simulink model "Yaw_EV_4WD"  (Simulink 8.8)
settings: Solver=ode45  StartTime=0  StopTime=10  FixedStep=0.002  RelTol=1e-3  AbsTol=1e-6
libraries: Solver_SF x1
settings Model: Creator=ywata  LastModifiedBy=mkhan  ExtModeTrigMode=oneshot  ExtModeArmWhenConnect=off
settings DataIOCC: LimitDataPoints=off  SignalLoggingName=sigsOut
settings OptimizationCC: BooleanDataType=off  ExpressionDepthLimit=2147483647
settings DebuggingCC: SaveWithParameterizedLinksMsg=none  SignalResolutionControl=TryResolveAllWithWarning  MultiTaskDSMMsg=warning  MultiTaskCondExecSysMsg=none  SFExecutionAtInitializationDiag=warning
settings HardwareCC: TargetUnknown=on
settings RTWCC: TemplateMakefile=grt_vc.tmf
settings ConfigComp: CovSFcnEnable=off

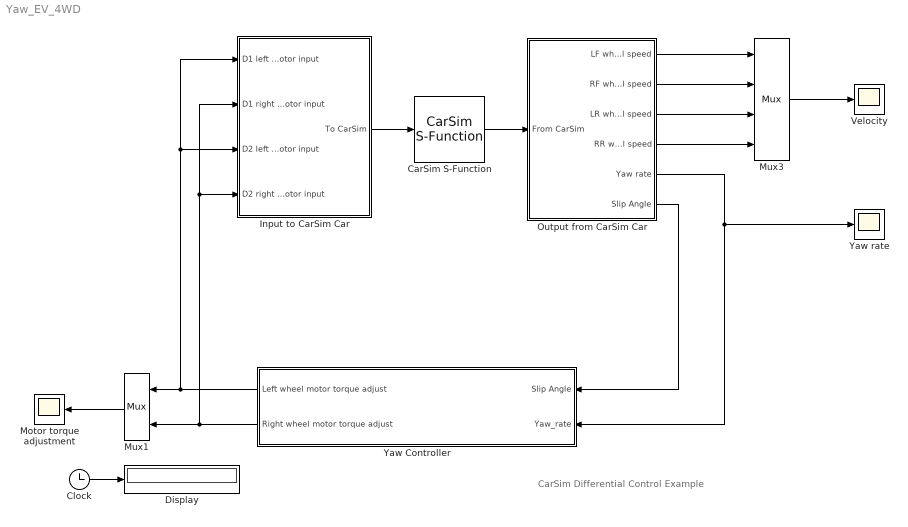
== system Yaw_EV_4WD ==
  note: CarSim Differential Control Example
  CarSim S-Function : Solver_SF/CarSim S-Function  Priority=1  SIMFILE=simfile.sim  Run_RTs=off  vs_state_ind=Run  StopMode_ind=Vehicle Model
  Clock : Clock
  Display : Display
      settings: Format=bank  Decimation=100
  Input to CarSim Car : Subsystem
  Motor torque adjustment : Scope
  Mux1 : Mux  Inputs=2
  Mux3 : Mux
  Output from CarSim Car : Subsystem
  Velocity : Scope
  Yaw Controller : Subsystem  mask{YAW=0.06, CONTROL=25, MAX_TORQUE=300}
      mask prompts: YAW "Yaw Control Gain (-)"; CONTROL "Control Gain (-)"; MAX_TORQUE "Maximum control torque (N)"
  Yaw rate : Scope
  wires:
  CarSim S-Function/1 -> Output from CarSim Car/1(From CarSim)
  Input to CarSim Car/1(To CarSim) -> CarSim S-Function/1
  Yaw Controller/1(Left wheel motor torque adjust) -> Mux1/1, Input to CarSim Car/3(D2 left motor input), Input to CarSim Car/1(D1 left motor input)
  Yaw Controller/2(Right wheel motor torque adjust) -> Input to CarSim Car/2(D1 right motor input), Input to CarSim Car/4(D2 right motor input), Mux1/2
  Clock/1 -> Display/1
  Mux3/1 -> Velocity/1
  Output from CarSim Car/6(Slip Angle) -> Yaw Controller/1(Slip Angle)
  Output from CarSim Car/5(Yaw rate) -> Yaw Controller/2(Yaw_rate), Yaw rate/1
  Output from CarSim Car/1(LF wheel speed) -> Mux3/1
  Output from CarSim Car/2(RF wheel speed) -> Mux3/2
  Output from CarSim Car/3(LR wheel speed) -> Mux3/3
  Output from CarSim Car/4(RR wheel speed) -> Mux3/4
  Mux1/1 -> Motor torque adjustment/1

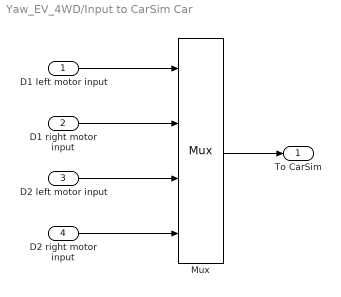
== system Yaw_EV_4WD/Input to CarSim Car ==
  D1 left motor input : Inport
  D1 right motor input : Inport  Port=2
  D2 left motor input : Inport  Port=3
  D2 right motor input : Inport  Port=4
  Mux : Mux
  To CarSim : Outport
  wires:
  Mux/1 -> To CarSim/1
  D2 right motor input/1 -> Mux/4
  D2 left motor input/1 -> Mux/3
  D1 left motor input/1 -> Mux/1
  D1 right motor input/1 -> Mux/2

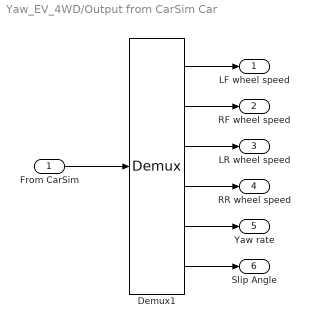
== system Yaw_EV_4WD/Output from CarSim Car ==
  From CarSim : Inport
  Demux1 : Demux  Outputs=6
      settings: DisplayOption=none
  LF wheel speed : Outport
  RF wheel speed : Outport  Port=2
  LR wheel speed : Outport  Port=3
  RR wheel speed : Outport  Port=4
  Yaw rate : Outport  Port=5
  Slip Angle : Outport  Port=6
  wires:
  From CarSim/1 -> Demux1/1
  Demux1/1 -> LF wheel speed/1
  Demux1/2 -> RF wheel speed/1
  Demux1/3 -> LR wheel speed/1
  Demux1/4 -> RR wheel speed/1
  Demux1/5 -> Yaw rate/1
  Demux1/6 -> Slip Angle/1

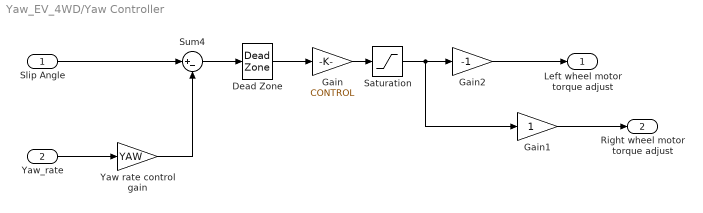
== system Yaw_EV_4WD/Yaw Controller ==
  Slip Angle : Inport
  Yaw_rate : Inport  Port=2
  Dead Zone : DeadZone  SaturateOnIntegerOverflow=on
  Gain : Gain  Gain=CONTROL  SaturateOnIntegerOverflow=on  OutDataTypeStr=Inherit: Same as input  ParamDataTypeStr=Inherit: Same as input
  Gain1 : Gain  SaturateOnIntegerOverflow=on  OutDataTypeStr=Inherit: Same as input  ParamDataTypeStr=Inherit: Same as input
  Gain2 : Gain  Gain=-1  SaturateOnIntegerOverflow=on  OutDataTypeStr=Inherit: Same as input  ParamDataTypeStr=Inherit: Same as input
  Saturation : Saturate  UpperLimit=MAX_TORQUE  LowerLimit=-MAX_TORQUE
  Sum4 : Sum  Inputs=|+-  InputSameDT=on  SaturateOnIntegerOverflow=on  OutDataTypeStr=Inherit: Same as first input
  Yaw rate control gain : Gain  Gain=YAW  SaturateOnIntegerOverflow=on  OutDataTypeStr=Inherit: Same as input  ParamDataTypeStr=Inherit: Same as input
  Left wheel motor torque adjust : Outport
  Right wheel motor torque adjust : Outport  Port=2
  wires:
  Yaw rate control gain/1 -> Sum4/2
  Yaw_rate/1 -> Yaw rate control gain/1
  Dead Zone/1 -> Gain/1
  Sum4/1 -> Dead Zone/1
  Gain/1 -> Saturation/1
  Gain1/1 -> Right wheel motor torque adjust/1
  Slip Angle/1 -> Sum4/1
  Gain2/1 -> Left wheel motor torque adjust/1
  Saturation/1 -> Gain1/1, Gain2/1
